simulink model "classwork_transfer"  (R2020a)
settings: Solver=VariableStepAuto  StartTime=0.0  StopTime=10.0  RelTol=1e-3
settings Model: Creator=surya  LastModifiedBy=surya

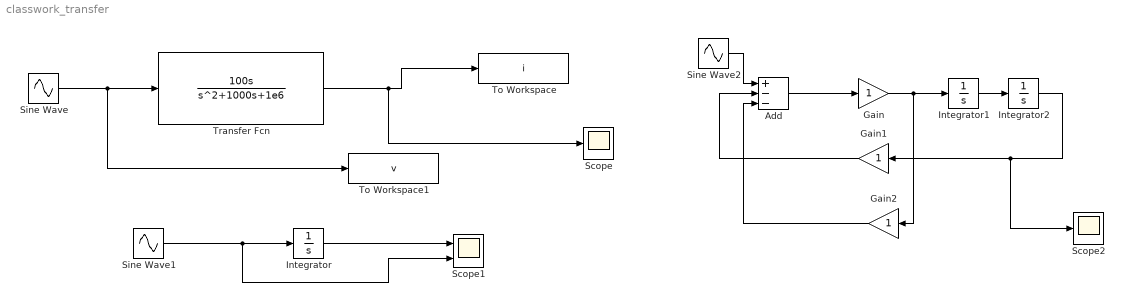
== system classwork_transfer ==
  Add : Sum  Inputs=+--
  Gain : Gain
  Gain1 : Gain
  Gain2 : Gain
  Integrator : Integrator  InitialCondition=-1
  Integrator1 : Integrator
  Integrator2 : Integrator
  Scope : Scope
  Scope1 : Scope  NumInputPorts=2
  Scope2 : Scope
  Sine Wave : Sin  SampleTime=0
  Sine Wave1 : Sin  Amplitude=3  Frequency=2  SampleTime=0
  Sine Wave2 : Sin  Amplitude=3  Frequency=2  SampleTime=0
  To Workspace : ToWorkspace  VariableName=i  SaveFormat=Timeseries  SampleTime=-1
  To Workspace1 : ToWorkspace  VariableName=v  SaveFormat=Timeseries  SampleTime=-1
  Transfer Fcn : TransferFcn  Numerator=[100 0]  Denominator=[1 1000 1e6]
  wires:
  Sine Wave/1 -> To Workspace1/1, Transfer Fcn/1
  Transfer Fcn/1 -> Scope/1, To Workspace/1
  Integrator/1 -> Scope1/1
  Sine Wave1/1 -> Scope1/2, Integrator/1
  Add/1 -> Gain/1
  Gain/1 -> Gain2/1, Integrator1/1
  Integrator1/1 -> Integrator2/1
  Integrator2/1 -> Scope2/1, Gain1/1
  Gain2/1 -> Add/3
  Gain1/1 -> Add/2
  Sine Wave2/1 -> Add/1
